simulink model "avg_speed_24a"  (R2024a)
settings: Solver=FixedStepDiscrete  StartTime=0.0  StopTime=10.0  FixedStep=0.01  RelTol=1e-3
model workspace (MAT data in the model file):
  threshold = Simulink.Parameter
  threshold.Value = 30
  threshold.Complexity = 'real'
  threshold.Dimensions = [1 1]
  threshold.DataType = 'single'
settings Model: Creator=developer  LastModifiedBy=developer
settings OptimizationCC: DefaultParameterBehavior=Inlined  EnhancedBackFolding=on  PassReuseOutputArgsAs=Individual arguments  ZeroExternalMemoryAtStartup=off  ZeroInternalMemoryAtStartup=off  OptimizeBlockOrder=speed  DifferentSizesBufferReuse=on  OptimizationCustomize=off  EfficientTunableParamExpr=on
settings DebuggingCC: ParameterTunabilityLossMsg=error  BusObjectLabelMismatch=error
settings SFSimCC: MATLABDynamicMemAlloc=off
settings RTWCC: Description=Embedded Coder  SystemTargetFile=ert.tlc  TemplateMakefile=ert_default_tmf  GPUComputeCapability=3.5
settings CodeAppCC: ForceParamTrailComments=on  IgnoreCustomStorageClasses=off  OperatorAnnotations=on  SimulinkDataObjDesc=on  SFDataObjDesc=on  InsertBlockDesc=on
settings ERTTargetCC: TargetLangStandard=C99 (ISO)  GenerateSampleERTMain=on  InlinedParameterPlacement=NonHierarchical  ERTCustomFileTemplate=example_file_process.tlc

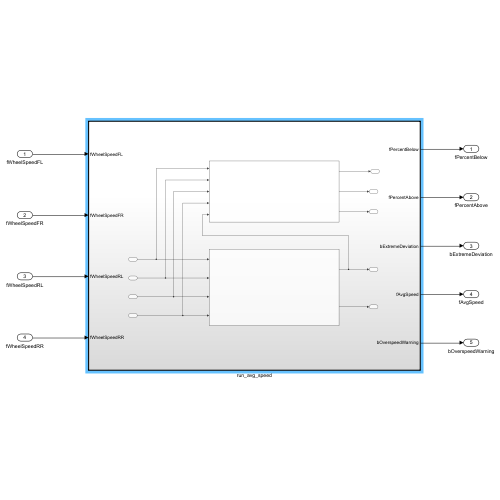
[thumbnail: Simulink's stored preview of the top-level diagram]
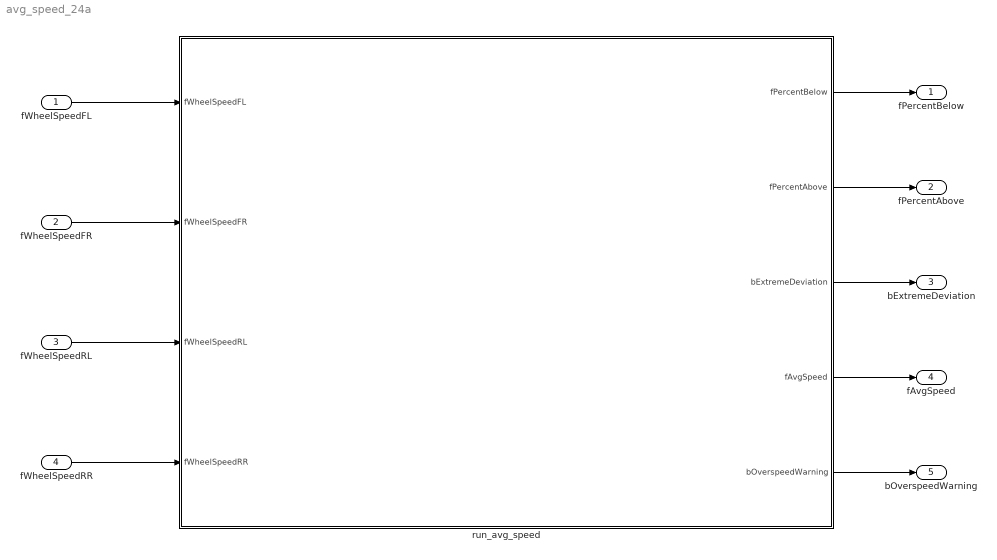
== system avg_speed_24a ==
  fWheelSpeedFL : Inport
  fWheelSpeedFR : Inport  Port=2
  fWheelSpeedRL : Inport  Port=3
  fWheelSpeedRR : Inport  Port=4
  run_avg_speed : Subsystem  TreatAsAtomicUnit=on
  fPercentBelow : Outport
  fPercentAbove : Outport  Port=2
  bExtremeDeviation : Outport  Port=3
  fAvgSpeed : Outport  Port=4
  bOverspeedWarning : Outport  Port=5
  wires:
  run_avg_speed/4(fAvgSpeed) -> fAvgSpeed/1
  run_avg_speed/3(bExtremeDeviation) -> bExtremeDeviation/1
  run_avg_speed/2(fPercentAbove) -> fPercentAbove/1
  fWheelSpeedFL/1 -> run_avg_speed/1(fWheelSpeedFL)
  fWheelSpeedFR/1 -> run_avg_speed/2(fWheelSpeedFR)
  fWheelSpeedRL/1 -> run_avg_speed/3(fWheelSpeedRL)
  fWheelSpeedRR/1 -> run_avg_speed/4(fWheelSpeedRR)
  run_avg_speed/1(fPercentBelow) -> fPercentBelow/1
  run_avg_speed/5(bOverspeedWarning) -> bOverspeedWarning/1

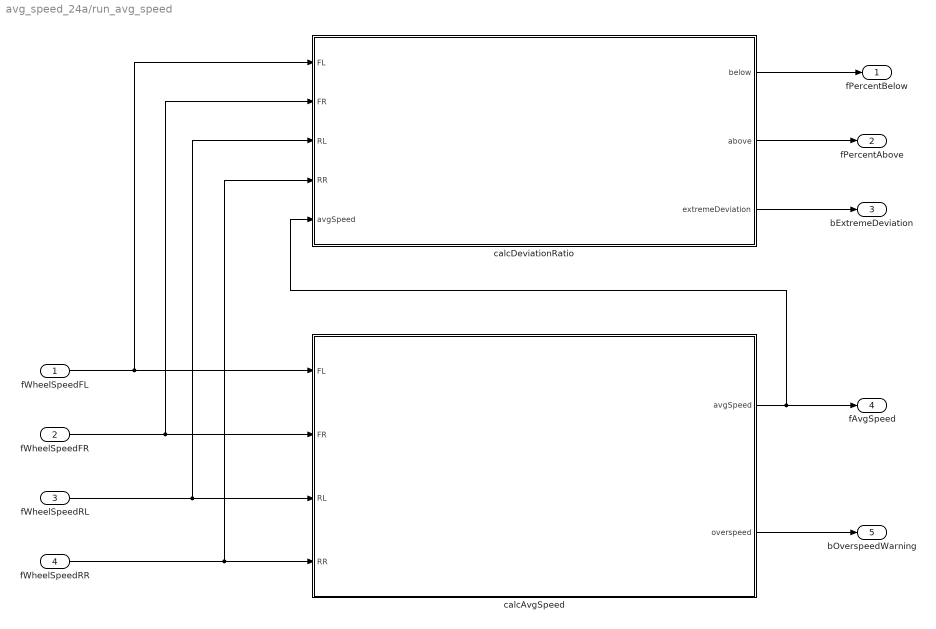
== system avg_speed_24a/run_avg_speed ==
  fWheelSpeedFL : Inport
  fWheelSpeedFR : Inport  Port=2
  fWheelSpeedRL : Inport  Port=3
  fWheelSpeedRR : Inport  Port=4
  calcAvgSpeed : Subsystem  TreatAsAtomicUnit=on
  calcDeviationRatio : Subsystem  TreatAsAtomicUnit=on
  fPercentBelow : Outport
  fPercentAbove : Outport  Port=2
  bExtremeDeviation : Outport  Port=3
  fAvgSpeed : Outport  Port=4
  bOverspeedWarning : Outport  Port=5
  wires:
  fWheelSpeedRR/1 -> calcAvgSpeed/4(RR), calcDeviationRatio/4(RR)
  fWheelSpeedFL/1 -> calcDeviationRatio/1(FL), calcAvgSpeed/1(FL)
  fWheelSpeedRL/1 -> calcAvgSpeed/3(RL), calcDeviationRatio/3(RL)
  calcAvgSpeed/2(overspeed) -> bOverspeedWarning/1
  fWheelSpeedFR/1 -> calcAvgSpeed/2(FR), calcDeviationRatio/2(FR)
  calcDeviationRatio/2(above) -> fPercentAbove/1
  calcAvgSpeed/1(avgSpeed) -> fAvgSpeed/1, calcDeviationRatio/5(avgSpeed)
  calcDeviationRatio/1(below) -> fPercentBelow/1
  calcDeviationRatio/3(extremeDeviation) -> bExtremeDeviation/1

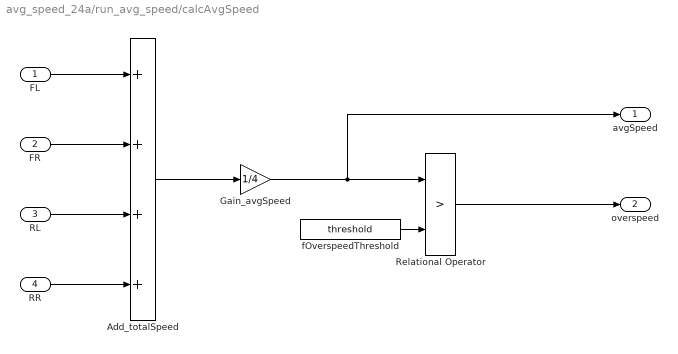
== system avg_speed_24a/run_avg_speed/calcAvgSpeed ==
  FL : Inport
  FR : Inport  Port=2
  RL : Inport  Port=3
  RR : Inport  Port=4
  Add_totalSpeed : Sum  Inputs=++++
  Gain_avgSpeed : Gain  Gain=1/4
  Relational Operator : RelationalOperator  Operator=>  OutDataTypeStr=boolean  RndMeth=Simplest  InputSameDT=off
  fOverspeedThreshold : Constant  Value=threshold
  avgSpeed : Outport
  overspeed : Outport  Port=2
  wires:
  fOverspeedThreshold/1 -> Relational Operator/2
  Gain_avgSpeed/1 -> avgSpeed/1, Relational Operator/1
  RL/1 -> Add_totalSpeed/3
  FR/1 -> Add_totalSpeed/2
  Add_totalSpeed/1 -> Gain_avgSpeed/1
  Relational Operator/1 -> overspeed/1
  RR/1 -> Add_totalSpeed/4
  FL/1 -> Add_totalSpeed/1

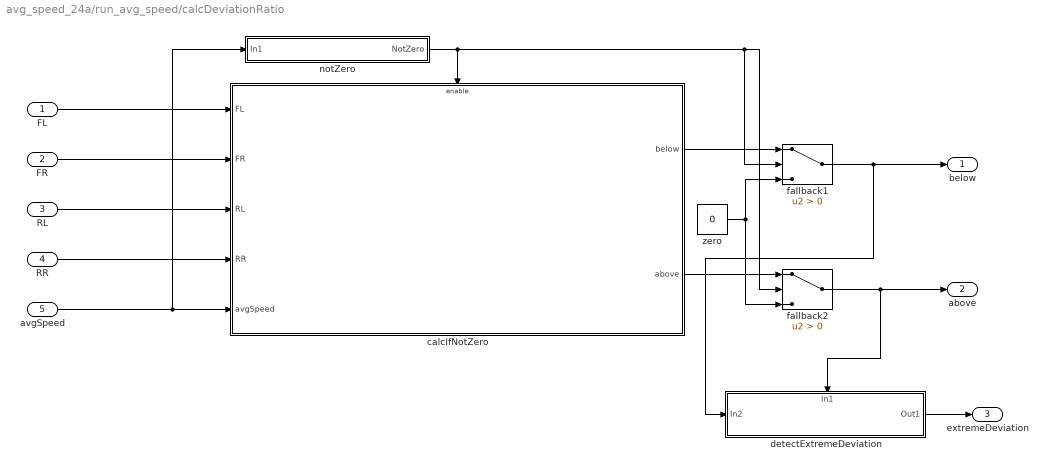
== system avg_speed_24a/run_avg_speed/calcDeviationRatio ==
  FL : Inport
  FR : Inport  Port=2
  RL : Inport  Port=3
  RR : Inport  Port=4
  avgSpeed : Inport  Port=5
  calcIfNotZero : Subsystem
      settings: RTWSystemCode=Nonreusable function  RTWFcnNameOpts=Use subsystem name
  detectExtremeDeviation : Subsystem
      settings: PortSchema="{\"entries\":[{\"content\":{\"sides\":[{\"content\":{\"connectorIds\":[\"In1\"]},\"type\":\"ConnectorPlacement.EquallySpacedRectSide\",\"uuid\":\"583db5ef-c387-4867-871e-9235f7e32af7\"},{\"content\":{\"connectorIds\":[\"Out1\"],\"side\":\"RIGHT\"},\"type\":\"ConnectorPlacement.EquallySpacedRectSide\",\"uuid\":\"84949f04-6f07-4642-b15e-054c50b68494\"},{\"content\":{\"connectorIds\":[\"In2\"],\"side\":\"TOP\"},\"type\":\"ConnectorPlacement.EquallySpacedRectSide\",\"uuid\":\"edb4fd78-6f55-41c1-a847-16b80f55a85f\"}]},\"type\":\"ConnectorPlacement.EquallySpacedConnector\",\"uuid\":\"09867930-2174-41af-bc9c-a8e1d1d345d4\"}],\"packageUris\":[\"http://schema.mathworks.com/mf0/Connector/R2020b\"],\"version\":\"1.0\"}"
  fallback1 : Switch  Criteria=u2 > Threshold  SaturateOnIntegerOverflow=off  InputSameDT=off
  fallback2 : Switch  Criteria=u2 > Threshold  SaturateOnIntegerOverflow=off  InputSameDT=off
  notZero : Subsystem
  zero : Constant  Value=0
  below : Outport
  above : Outport  Port=2
  extremeDeviation : Outport  Port=3
  wires:
  notZero/1(NotZero) -> calcIfNotZero/Enable, fallback2/2, fallback1/2
  RR/1 -> calcIfNotZero/4(RR)
  calcIfNotZero/1(below) -> fallback1/1
  calcIfNotZero/2(above) -> fallback2/1
  avgSpeed/1 -> calcIfNotZero/5(avgSpeed), notZero/1(In1)
  FR/1 -> calcIfNotZero/2(FR)
  zero/1 -> fallback2/3, fallback1/3
  FL/1 -> calcIfNotZero/1(FL)
  RL/1 -> calcIfNotZero/3(RL)
  fallback1/1 -> detectExtremeDeviation/1(In2), below/1
  detectExtremeDeviation/1(Out1) -> extremeDeviation/1
  fallback2/1 -> detectExtremeDeviation/2(In1), above/1

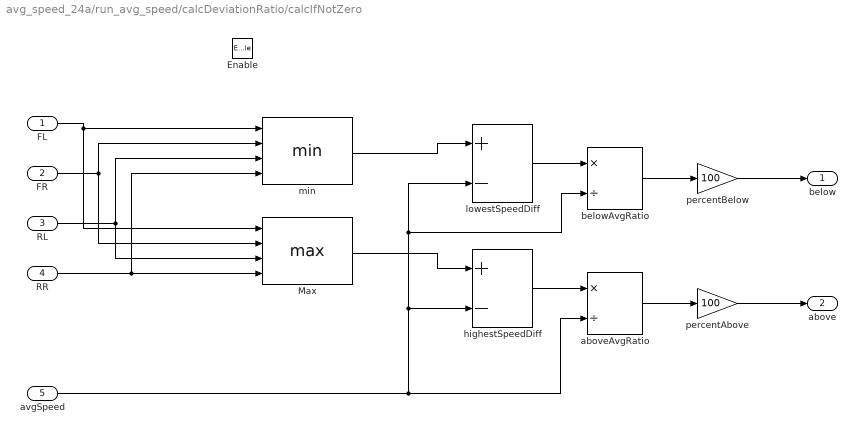
== system avg_speed_24a/run_avg_speed/calcDeviationRatio/calcIfNotZero ==
  FL : Inport
  FR : Inport  Port=2
  RL : Inport  Port=3
  RR : Inport  Port=4
  avgSpeed : Inport  Port=5
  Enable : EnablePort
  Max : MinMax  Function=max  Inputs=4
  aboveAvgRatio : Product  Inputs=*/
  belowAvgRatio : Product  Inputs=*/
  highestSpeedDiff : Sum  Inputs=+-
  lowestSpeedDiff : Sum  Inputs=+-
  min : MinMax  Inputs=4
  percentAbove : Gain  Gain=100
  percentBelow : Gain  Gain=100
  below : Outport
  above : Outport  Port=2
  wires:
  min/1 -> lowestSpeedDiff/1
  RL/1 -> min/3, Max/3
  FL/1 -> Max/1, min/1
  RR/1 -> min/4, Max/4
  FR/1 -> Max/2, min/2
  percentAbove/1 -> above/1
  Max/1 -> highestSpeedDiff/1
  lowestSpeedDiff/1 -> belowAvgRatio/1
  belowAvgRatio/1 -> percentBelow/1
  highestSpeedDiff/1 -> aboveAvgRatio/1
  aboveAvgRatio/1 -> percentAbove/1
  avgSpeed/1 -> aboveAvgRatio/2, belowAvgRatio/2, lowestSpeedDiff/2, highestSpeedDiff/2
  percentBelow/1 -> below/1

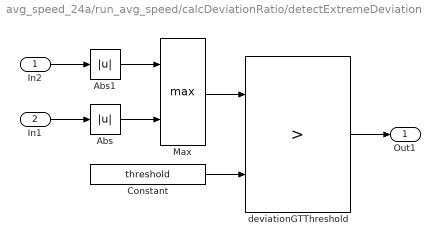
== system avg_speed_24a/run_avg_speed/calcDeviationRatio/detectExtremeDeviation ==
  In2 : Inport
  In1 : Inport  Port=2
  Abs : Abs  SaturateOnIntegerOverflow=off
  Abs1 : Abs  SaturateOnIntegerOverflow=off
  Constant : Constant  Value=threshold
  Max : MinMax  Function=max  Inputs=2
  deviationGTThreshold : RelationalOperator  Operator=>  OutDataTypeStr=boolean  RndMeth=Simplest  InputSameDT=off
  Out1 : Outport
  wires:
  In1/1 -> Abs/1
  In2/1 -> Abs1/1
  Constant/1 -> deviationGTThreshold/2
  Abs1/1 -> Max/1
  Abs/1 -> Max/2
  Max/1 -> deviationGTThreshold/1
  deviationGTThreshold/1 -> Out1/1

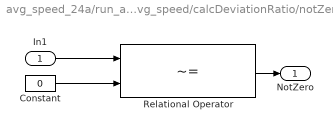
== system avg_speed_24a/run_avg_speed/calcDeviationRatio/notZero ==
  In1 : Inport
  Constant : Constant  Value=0
  Relational Operator : RelationalOperator  Operator=~=  OutDataTypeStr=boolean  RndMeth=Simplest  InputSameDT=off
  NotZero : Outport
  wires:
  Constant/1 -> Relational Operator/2
  Relational Operator/1 -> NotZero/1
  In1/1 -> Relational Operator/1
